simulink model "gab"  (R2018b)
settings: Solver=ode45  StartTime=0.0  StopTime=30000  RelTol=1e-3
values from neighbouring files (symbols this model uses):
  M = k3+k34*k4/sqrt(k34^2+k4^2)    [Lin_Analitica.m]    (also in ident_master.m = 1; identif.m = 2)
  PO = 12    [ident_master.m]    (also in identif.m = 10)
  qmax = 120    [para4nl.m]
  qmin = -120    [para4nl.m]
settings Model: Creator=root  LastModifiedBy=root

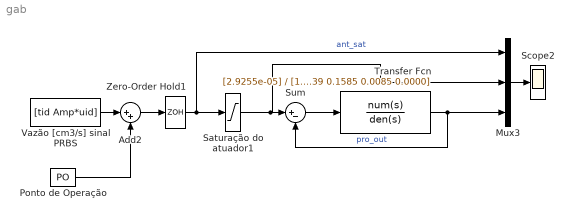
== system gab ==
  Add2 : Sum  Inputs=|++
  Mux3 : Mux  Inputs=3
  "Ponto de Operação " : Constant  Value=PO
  Saturação do atuador1 : Saturate  UpperLimit=qmax  LowerLimit=qmin
  Scope2 : Scope
  Sum : Sum  Inputs=|+-
  Transfer Fcn : TransferFcn  Numerator=[2.9255e-05]  Denominator=[1.0000 0.7639 0.1585 0.0085 0.0000]
  Vazão [cm3/s] sinal PRBS : FromWorkspace  VariableName=[tid Amp*uid]  SampleTime=10  Interpolate=off  OutputAfterFinalValue=Holding final value
  Zero-Order Hold1 : ZeroOrderHold  SampleTime=M
  wires:
  "Ponto de Operação "/1 -> Add2/2
  Saturação do atuador1/1 -> Sum/1, Mux3/2
  Vazão [cm3/s] sinal PRBS/1 -> Add2/1
  Zero-Order Hold1/1 -> Mux3/1, Saturação do atuador1/1  "ant_sat"
  Mux3/1 -> Scope2/1
  Add2/1 -> Zero-Order Hold1/1
  Transfer Fcn/1 -> Sum/2, Mux3/3  "pro_out"
  Sum/1 -> Transfer Fcn/1
